simulink model "Isooffboard_SSC"  (R2025b)
settings: Solver=VariableStepAuto  StartTime=0.0  StopTime=0.5  RelTol=1e-3
undefined symbols (not defined in the file): V_ref_isolated
libraries: fl_lib x73, nesl_utility x29, ee_lib x9, simulink x3, eeTransforms x2, batteryecm_lib x1, eeSinusoidalMeasurementV2 x1
(part 2 of 3)

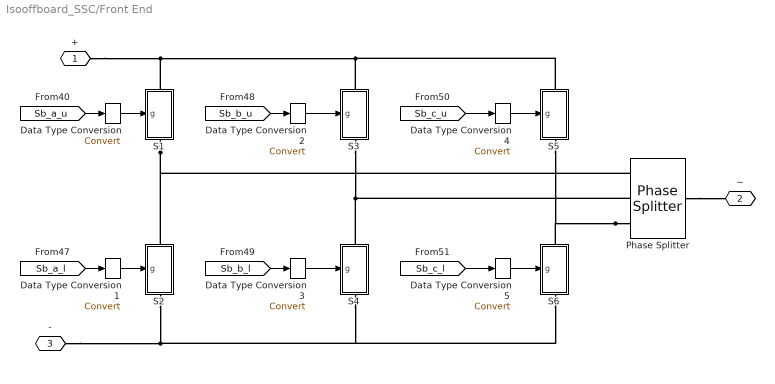
== system Isooffboard_SSC/Front End ==
  Data Type Conversion{,1..5} (6 alike) : DataTypeConversion  SaturateOnIntegerOverflow=off  RndMeth=Floor
  Phase Splitter : ee_lib/Connectors & References/Phase Splitter
  S1 : Subsystem
      settings: PortSchema="{\"entries\":[{\"content\":{\"sides\":[{\"content\":{\"connectorIds\":[\"In1\"]},\"type\":\"ConnectorPlacement.EquallySpacedRectSide\",\"uuid\":\"4868c43b-8f86-4e2f-a4da-367c2e17d6e4\"},{\"content\":{\"side\":\"RIGHT\"},\"type\":\"ConnectorPlacement.EquallySpacedRectSide\",\"uuid\":\"ebe9b5ec-833b-4a08-98e5-ff684cd7afcb\"},{\"content\":{\"connectorIds\":[\"LConn1\"],\"side\":\"TOP\"},\"type\":\"ConnectorPlacement.EquallySpacedRectSide\",\"uuid\":\"c72df866-8baa-41a8-9bb1-42a4a1fdee71\"},{\"content\":{\"connectorIds\":[\"RConn1\"],\"side\":\"BOTTOM\"},\"type\":\"ConnectorPlacement.EquallySpacedRectSide\",\"uuid\":\"3a9867c5-1563-48cb-a4f4-92deec85fd3d\"}]},\"type\":\"ConnectorPlacement.EquallySpacedConnector\",\"uuid\":\"206e0d7b-1d35-45e7-9c4c-8a6f9fe9dc79\"}],\"packageUris\":[\"http://schema.mathworks.com/mf0/Connector/R2020b\"],\"version\":\"1.0\"}"
  S2 : Subsystem
      settings: PortSchema="{\"entries\":[{\"content\":{\"sides\":[{\"content\":{\"connectorIds\":[\"In1\"]},\"type\":\"ConnectorPlacement.EquallySpacedRectSide\",\"uuid\":\"4868c43b-8f86-4e2f-a4da-367c2e17d6e4\"},{\"content\":{\"side\":\"RIGHT\"},\"type\":\"ConnectorPlacement.EquallySpacedRectSide\",\"uuid\":\"ebe9b5ec-833b-4a08-98e5-ff684cd7afcb\"},{\"content\":{\"connectorIds\":[\"LConn1\"],\"side\":\"TOP\"},\"type\":\"ConnectorPlacement.EquallySpacedRectSide\",\"uuid\":\"c72df866-8baa-41a8-9bb1-42a4a1fdee71\"},{\"content\":{\"connectorIds\":[\"RConn1\"],\"side\":\"BOTTOM\"},\"type\":\"ConnectorPlacement.EquallySpacedRectSide\",\"uuid\":\"3a9867c5-1563-48cb-a4f4-92deec85fd3d\"}]},\"type\":\"ConnectorPlacement.EquallySpacedConnector\",\"uuid\":\"206e0d7b-1d35-45e7-9c4c-8a6f9fe9dc79\"}],\"packageUris\":[\"http://schema.mathworks.com/mf0/Connector/R2020b\"],\"version\":\"1.0\"}"
  S3 : Subsystem
      settings: PortSchema="{\"entries\":[{\"content\":{\"sides\":[{\"content\":{\"connectorIds\":[\"In1\"]},\"type\":\"ConnectorPlacement.EquallySpacedRectSide\",\"uuid\":\"4868c43b-8f86-4e2f-a4da-367c2e17d6e4\"},{\"content\":{\"side\":\"RIGHT\"},\"type\":\"ConnectorPlacement.EquallySpacedRectSide\",\"uuid\":\"ebe9b5ec-833b-4a08-98e5-ff684cd7afcb\"},{\"content\":{\"connectorIds\":[\"LConn1\"],\"side\":\"TOP\"},\"type\":\"ConnectorPlacement.EquallySpacedRectSide\",\"uuid\":\"c72df866-8baa-41a8-9bb1-42a4a1fdee71\"},{\"content\":{\"connectorIds\":[\"RConn1\"],\"side\":\"BOTTOM\"},\"type\":\"ConnectorPlacement.EquallySpacedRectSide\",\"uuid\":\"3a9867c5-1563-48cb-a4f4-92deec85fd3d\"}]},\"type\":\"ConnectorPlacement.EquallySpacedConnector\",\"uuid\":\"206e0d7b-1d35-45e7-9c4c-8a6f9fe9dc79\"}],\"packageUris\":[\"http://schema.mathworks.com/mf0/Connector/R2020b\"],\"version\":\"1.0\"}"
  S4 : Subsystem
      settings: PortSchema="{\"entries\":[{\"content\":{\"sides\":[{\"content\":{\"connectorIds\":[\"In1\"]},\"type\":\"ConnectorPlacement.EquallySpacedRectSide\",\"uuid\":\"4868c43b-8f86-4e2f-a4da-367c2e17d6e4\"},{\"content\":{\"side\":\"RIGHT\"},\"type\":\"ConnectorPlacement.EquallySpacedRectSide\",\"uuid\":\"ebe9b5ec-833b-4a08-98e5-ff684cd7afcb\"},{\"content\":{\"connectorIds\":[\"LConn1\"],\"side\":\"TOP\"},\"type\":\"ConnectorPlacement.EquallySpacedRectSide\",\"uuid\":\"c72df866-8baa-41a8-9bb1-42a4a1fdee71\"},{\"content\":{\"connectorIds\":[\"RConn1\"],\"side\":\"BOTTOM\"},\"type\":\"ConnectorPlacement.EquallySpacedRectSide\",\"uuid\":\"3a9867c5-1563-48cb-a4f4-92deec85fd3d\"}]},\"type\":\"ConnectorPlacement.EquallySpacedConnector\",\"uuid\":\"206e0d7b-1d35-45e7-9c4c-8a6f9fe9dc79\"}],\"packageUris\":[\"http://schema.mathworks.com/mf0/Connector/R2020b\"],\"version\":\"1.0\"}"
  S5 : Subsystem
      settings: PortSchema="{\"entries\":[{\"content\":{\"sides\":[{\"content\":{\"connectorIds\":[\"In1\"]},\"type\":\"ConnectorPlacement.EquallySpacedRectSide\",\"uuid\":\"4868c43b-8f86-4e2f-a4da-367c2e17d6e4\"},{\"content\":{\"side\":\"RIGHT\"},\"type\":\"ConnectorPlacement.EquallySpacedRectSide\",\"uuid\":\"ebe9b5ec-833b-4a08-98e5-ff684cd7afcb\"},{\"content\":{\"connectorIds\":[\"LConn1\"],\"side\":\"TOP\"},\"type\":\"ConnectorPlacement.EquallySpacedRectSide\",\"uuid\":\"c72df866-8baa-41a8-9bb1-42a4a1fdee71\"},{\"content\":{\"connectorIds\":[\"RConn1\"],\"side\":\"BOTTOM\"},\"type\":\"ConnectorPlacement.EquallySpacedRectSide\",\"uuid\":\"3a9867c5-1563-48cb-a4f4-92deec85fd3d\"}]},\"type\":\"ConnectorPlacement.EquallySpacedConnector\",\"uuid\":\"206e0d7b-1d35-45e7-9c4c-8a6f9fe9dc79\"}],\"packageUris\":[\"http://schema.mathworks.com/mf0/Connector/R2020b\"],\"version\":\"1.0\"}"
  S6 : Subsystem
      settings: PortSchema="{\"entries\":[{\"content\":{\"sides\":[{\"content\":{\"connectorIds\":[\"In1\"]},\"type\":\"ConnectorPlacement.EquallySpacedRectSide\",\"uuid\":\"4868c43b-8f86-4e2f-a4da-367c2e17d6e4\"},{\"content\":{\"side\":\"RIGHT\"},\"type\":\"ConnectorPlacement.EquallySpacedRectSide\",\"uuid\":\"ebe9b5ec-833b-4a08-98e5-ff684cd7afcb\"},{\"content\":{\"connectorIds\":[\"LConn1\"],\"side\":\"TOP\"},\"type\":\"ConnectorPlacement.EquallySpacedRectSide\",\"uuid\":\"c72df866-8baa-41a8-9bb1-42a4a1fdee71\"},{\"content\":{\"connectorIds\":[\"RConn1\"],\"side\":\"BOTTOM\"},\"type\":\"ConnectorPlacement.EquallySpacedRectSide\",\"uuid\":\"3a9867c5-1563-48cb-a4f4-92deec85fd3d\"}]},\"type\":\"ConnectorPlacement.EquallySpacedConnector\",\"uuid\":\"206e0d7b-1d35-45e7-9c4c-8a6f9fe9dc79\"}],\"packageUris\":[\"http://schema.mathworks.com/mf0/Connector/R2020b\"],\"version\":\"1.0\"}"
  + : PMIOPort  Side=Right
  "~ " : PMIOPort  Port=2  Side=Left
  - : PMIOPort  Port=3  Side=Right
  wires:
  [Sb_c_l] -> Data Type Conversion5/1
  [Sb_b_l] -> Data Type Conversion3/1
  [Sb_a_l] -> Data Type Conversion1/1
  [Sb_a_u] -> Data Type Conversion/1
  [Sb_c_u] -> Data Type Conversion4/1
  [Sb_b_u] -> Data Type Conversion2/1
  Data Type Conversion/1 -> S1/1(g)
  Data Type Conversion1/1 -> S2/1(g)
  Data Type Conversion2/1 -> S3/1(g)
  Data Type Conversion3/1 -> S4/1(g)
  Data Type Conversion4/1 -> S5/1(g)
  Data Type Conversion5/1 -> S6/1(g)
  connections:
  S6/RConn1 -- S4/RConn1 -- S2/RConn1 -- -/RConn1
  S1/LConn1 -- S5/LConn1 -- S3/LConn1 -- +/RConn1
  Phase Splitter/RConn3 -- S6/LConn1 -- S5/RConn1
  Phase Splitter/RConn2 -- S4/LConn1 -- S3/RConn1
  S1/RConn1 -- S2/LConn1 -- Phase Splitter/RConn1
  Phase Splitter/LConn1 -- "~ "/RConn1

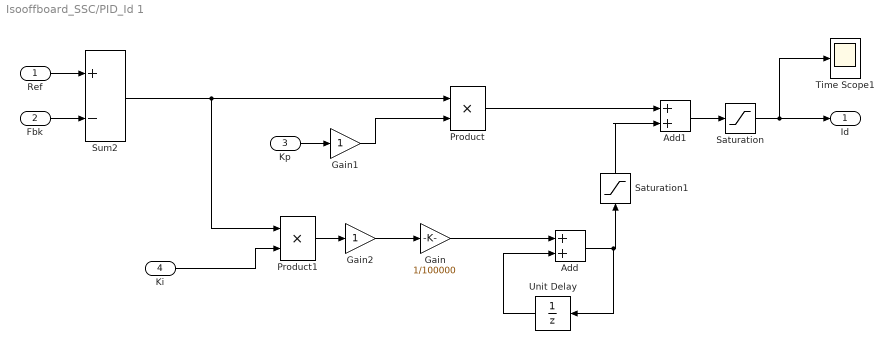
== system Isooffboard_SSC/PID_Id 1 ==
  Ref : Inport
  Fbk : Inport  Port=2
  Kp : Inport  Port=3
  Ki : Inport  Port=4
  Add : Sum
  Add1 : Sum
  Gain : Gain  Gain=1/100000
  Gain1 : Gain
  Gain2 : Gain
  Product : Product  OutDataTypeStr=Inherit: Same as first input
  Product1 : Product  OutDataTypeStr=Inherit: Same as first input
  Saturation : Saturate  UpperLimit=200  LowerLimit=-200  LinearizeAsGain=off  ZeroCross=off
  Saturation1 : Saturate  UpperLimit=200  LowerLimit=-200  LinearizeAsGain=off  ZeroCross=off
  Sum2 : Sum  Inputs=+-
  Time Scope1 : Scope
      settings: TimeUnits=Metric (based on Time Span)  ActiveDisplayYMinimum=-250  ActiveDisplayYMaximum=250  YLabel=Amplitude  DataLoggingVariableName=ScopeData5
  Unit Delay : UnitDelay  SampleTime=-1  HasFrameUpgradeWarning=on
  Id : Outport
  wires:
  Sum2/1 -> Product1/1, Product/1
  Fbk/1 -> Sum2/2
  Ref/1 -> Sum2/1
  Product1/1 -> Gain2/1
  Add/1 -> Unit Delay/1, Saturation1/1
  Product/1 -> Add1/1
  Gain/1 -> Add/1
  Unit Delay/1 -> Add/2
  Kp/1 -> Gain1/1
  Ki/1 -> Product1/2
  Gain1/1 -> Product/2
  Gain2/1 -> Gain/1
  Add1/1 -> Saturation/1
  Saturation/1 -> Time Scope1/1, Id/1
  Saturation1/1 -> Add1/2

== system Isooffboard_SSC/PID_Id 2 ==
  Ref : Inport
  Fbk : Inport  Port=2
  Kp : Inport  Port=3
  Ki : Inport  Port=4
  Add : Sum
  Add1 : Sum
  Gain : Gain  Gain=1/100000
  Product : Product  OutDataTypeStr=Inherit: Same as first input
  Product1 : Product  OutDataTypeStr=Inherit: Same as first input
  Saturation : Saturate  UpperLimit=900  LowerLimit=-900  LinearizeAsGain=off  ZeroCross=off
  Saturation1 : Saturate  UpperLimit=900  LowerLimit=-900  ZeroCross=off
  Sum2 : Sum  Inputs=+-
  Time Scope1 : Scope
      settings: TimeUnits=Metric (based on Time Span)  ActiveDisplayYMinimum=-1125  ActiveDisplayYMaximum=1125  YLabel=Amplitude  DataLoggingVariableName=ScopeData5
  Unit Delay : UnitDelay  SampleTime=-1  HasFrameUpgradeWarning=on
  Ud : Outport
  wires:
  Add1/1 -> Saturation/1
  Sum2/1 -> Product1/1, Product/1
  Fbk/1 -> Sum2/2
  Ref/1 -> Sum2/1
  Kp/1 -> Product/2
  Ki/1 -> Product1/2
  Product1/1 -> Gain/1
  Add/1 -> Unit Delay/1, Saturation1/1
  Product/1 -> Add1/1
  Saturation/1 -> Time Scope1/1, Ud/1
  Gain/1 -> Add/1
  Unit Delay/1 -> Add/2
  Saturation1/1 -> Add1/2

== system Isooffboard_SSC/PID_Iq 3 ==
  Ref : Inport
  Fbk : Inport  Port=2
  Kp : Inport  Port=3
  Ki : Inport  Port=4
  Add : Sum
  Add1 : Sum
  Gain : Gain  Gain=1/100000
  Product : Product  OutDataTypeStr=Inherit: Same as first input
  Product1 : Product  OutDataTypeStr=Inherit: Same as first input
  Saturation : Saturate  UpperLimit=900  LowerLimit=-900  LinearizeAsGain=off  ZeroCross=off
  Saturation1 : Saturate  UpperLimit=900  LowerLimit=-900  LinearizeAsGain=off  ZeroCross=off
  Sum2 : Sum  Inputs=+-
  Time Scope1 : Scope
      settings: TimeUnits=Metric (based on Time Span)  ActiveDisplayYMinimum=-295.24637  ActiveDisplayYMaximum=1032.80515  YLabel=Amplitude  DataLoggingVariableName=ScopeData6
  Unit Delay : UnitDelay  SampleTime=-1  HasFrameUpgradeWarning=on
  Uq : Outport
  wires:
  Add1/1 -> Saturation/1
  Sum2/1 -> Product1/1, Product/1
  Fbk/1 -> Sum2/2
  Ref/1 -> Sum2/1
  Kp/1 -> Product/2
  Ki/1 -> Product1/2
  Product1/1 -> Gain/1
  Add/1 -> Unit Delay/1, Saturation1/1
  Product/1 -> Add1/1
  Gain/1 -> Add/1
  Unit Delay/1 -> Add/2
  Saturation/1 -> Time Scope1/1, Uq/1
  Saturation1/1 -> Add1/2

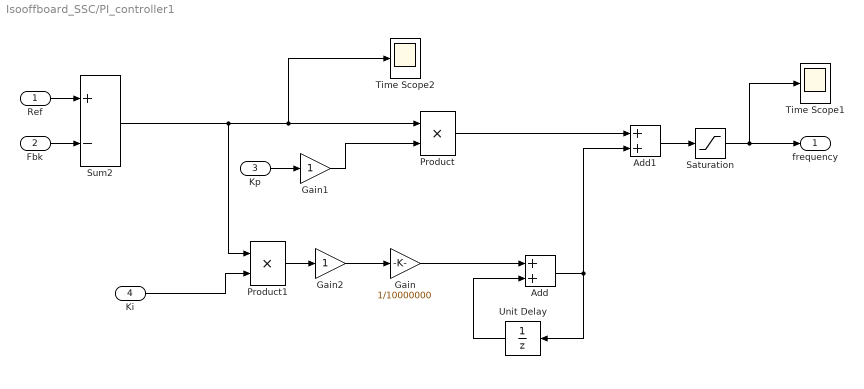
== system Isooffboard_SSC/PI_controller1 ==
  Ref : Inport
  Fbk : Inport  Port=2
  Kp : Inport  Port=3
  Ki : Inport  Port=4
  Add : Sum
  Add1 : Sum
  Gain : Gain  Gain=1/10000000
  Gain1 : Gain
  Gain2 : Gain
  Product : Product  OutDataTypeStr=Inherit: Same as first input
  Product1 : Product  OutDataTypeStr=Inherit: Same as first input
  Saturation : Saturate  UpperLimit=1  LowerLimit=0.5  LinearizeAsGain=off  ZeroCross=off
  Sum2 : Sum  Inputs=+-
  Time Scope1 : Scope
      settings: TimeUnits=Metric (based on Time Span)  ActiveDisplayYMinimum=0.4375  ActiveDisplayYMaximum=1.0625  YLabel=Amplitude  DataLoggingVariableName=ScopeData5
  Time Scope2 : Scope
      settings: TimeUnits=Metric (based on Time Span)  ActiveDisplayYMinimum=-48.22028  ActiveDisplayYMaximum=227.58003  YLabel=Amplitude  DataLoggingVariableName=ScopeData6
  Unit Delay : UnitDelay  InitialCondition=0.9  SampleTime=-1  HasFrameUpgradeWarning=on
  frequency : Outport
  wires:
  Fbk/1 -> Sum2/2
  Ref/1 -> Sum2/1
  Product1/1 -> Gain2/1
  Add/1 -> Unit Delay/1, Add1/2
  Product/1 -> Add1/1
  Gain/1 -> Add/1
  Unit Delay/1 -> Add/2
  Ki/1 -> Product1/2
  Gain2/1 -> Gain/1
  Add1/1 -> Saturation/1
  Saturation/1 -> Time Scope1/1, frequency/1
  Kp/1 -> Gain1/1
  Gain1/1 -> Product/2
  Sum2/1 -> Product1/1, Time Scope2/1, Product/1

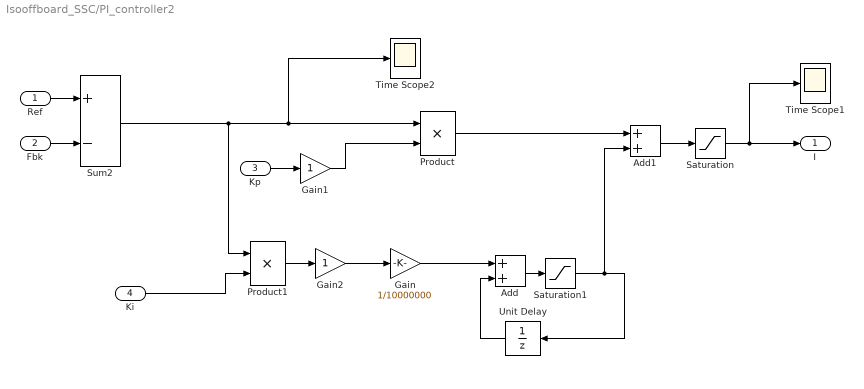
== system Isooffboard_SSC/PI_controller2 ==
  Ref : Inport
  Fbk : Inport  Port=2
  Kp : Inport  Port=3
  Ki : Inport  Port=4
  Add : Sum
  Add1 : Sum
  Gain : Gain  Gain=1/10000000
  Gain1 : Gain
  Gain2 : Gain
  Product : Product  OutDataTypeStr=Inherit: Same as first input
  Product1 : Product  OutDataTypeStr=Inherit: Same as first input
  Saturation : Saturate  UpperLimit=50  LowerLimit=-50  LinearizeAsGain=off  ZeroCross=off
  Saturation1 : Saturate  UpperLimit=50  LowerLimit=-50  LinearizeAsGain=off  ZeroCross=off
  Sum2 : Sum  Inputs=+-
  Time Scope1 : Scope
      settings: TimeUnits=Metric (based on Time Span)  ActiveDisplayYMinimum=-55.24132  ActiveDisplayYMaximum=61.69348  YLabel=Amplitude  DataLoggingVariableName=ScopeData5
  Time Scope2 : Scope
      settings: TimeUnits=Metric (based on Time Span)  ActiveDisplayYMinimum=-48.22028  ActiveDisplayYMaximum=227.58003  YLabel=Amplitude  DataLoggingVariableName=ScopeData6
  Unit Delay : UnitDelay  InitialCondition=0.9  SampleTime=-1  HasFrameUpgradeWarning=on
  I : Outport
  wires:
  Fbk/1 -> Sum2/2
  Ref/1 -> Sum2/1
  Product1/1 -> Gain2/1
  Product/1 -> Add1/1
  Gain/1 -> Add/1
  Unit Delay/1 -> Add/2
  Ki/1 -> Product1/2
  Gain2/1 -> Gain/1
  Add1/1 -> Saturation/1
  Saturation/1 -> Time Scope1/1, I/1
  Kp/1 -> Gain1/1
  Gain1/1 -> Product/2
  Sum2/1 -> Product1/1, Time Scope2/1, Product/1
  Add/1 -> Saturation1/1
  Saturation1/1 -> Add1/2, Unit Delay/1

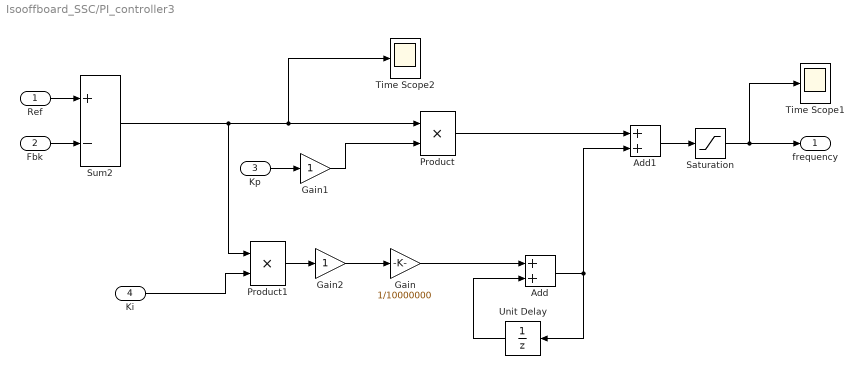
== system Isooffboard_SSC/PI_controller3 ==
  Ref : Inport
  Fbk : Inport  Port=2
  Kp : Inport  Port=3
  Ki : Inport  Port=4
  Add : Sum
  Add1 : Sum
  Gain : Gain  Gain=1/10000000
  Gain1 : Gain
  Gain2 : Gain
  Product : Product  OutDataTypeStr=Inherit: Same as first input
  Product1 : Product  OutDataTypeStr=Inherit: Same as first input
  Saturation : Saturate  UpperLimit=1  LowerLimit=0.5  LinearizeAsGain=off  ZeroCross=off
  Sum2 : Sum  Inputs=+-
  Time Scope1 : Scope
      settings: TimeUnits=Metric (based on Time Span)  ActiveDisplayYMinimum=0.4375  ActiveDisplayYMaximum=1.0625  YLabel=Amplitude  DataLoggingVariableName=ScopeData5
  Time Scope2 : Scope
      settings: TimeUnits=Metric (based on Time Span)  ActiveDisplayYMinimum=-48.22028  ActiveDisplayYMaximum=227.58003  YLabel=Amplitude  DataLoggingVariableName=ScopeData6
  Unit Delay : UnitDelay  InitialCondition=0.9  SampleTime=-1  HasFrameUpgradeWarning=on
  frequency : Outport
  wires:
  Fbk/1 -> Sum2/2
  Ref/1 -> Sum2/1
  Product1/1 -> Gain2/1
  Add/1 -> Unit Delay/1, Add1/2
  Product/1 -> Add1/1
  Gain/1 -> Add/1
  Unit Delay/1 -> Add/2
  Ki/1 -> Product1/2
  Gain2/1 -> Gain/1
  Add1/1 -> Saturation/1
  Saturation/1 -> Time Scope1/1, frequency/1
  Kp/1 -> Gain1/1
  Gain1/1 -> Product/2
  Sum2/1 -> Product1/1, Time Scope2/1, Product/1

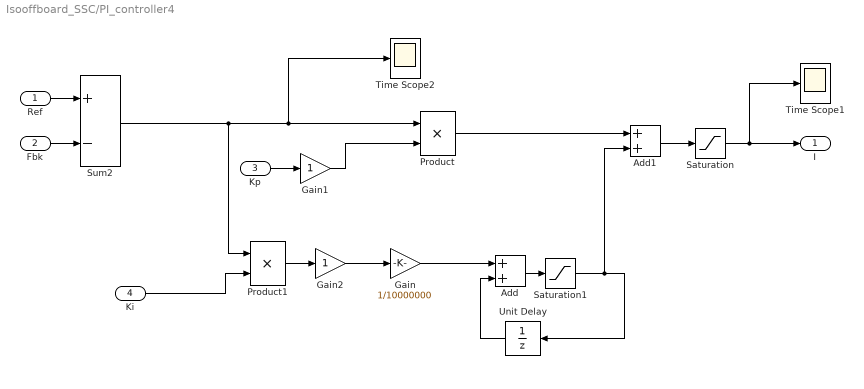
== system Isooffboard_SSC/PI_controller4 ==
  Ref : Inport
  Fbk : Inport  Port=2
  Kp : Inport  Port=3
  Ki : Inport  Port=4
  Add : Sum
  Add1 : Sum
  Gain : Gain  Gain=1/10000000
  Gain1 : Gain
  Gain2 : Gain
  Product : Product  OutDataTypeStr=Inherit: Same as first input
  Product1 : Product  OutDataTypeStr=Inherit: Same as first input
  Saturation : Saturate  UpperLimit=50  LowerLimit=-50  LinearizeAsGain=off  ZeroCross=off
  Saturation1 : Saturate  UpperLimit=50  LowerLimit=-50  LinearizeAsGain=off  ZeroCross=off
  Sum2 : Sum  Inputs=+-
  Time Scope1 : Scope
      settings: TimeUnits=Metric (based on Time Span)  ActiveDisplayYMinimum=-55.24132  ActiveDisplayYMaximum=61.69348  YLabel=Amplitude  DataLoggingVariableName=ScopeData5
  Time Scope2 : Scope
      settings: TimeUnits=Metric (based on Time Span)  ActiveDisplayYMinimum=-48.22028  ActiveDisplayYMaximum=227.58003  YLabel=Amplitude  DataLoggingVariableName=ScopeData6
  Unit Delay : UnitDelay  InitialCondition=0.9  SampleTime=-1  HasFrameUpgradeWarning=on
  I : Outport
  wires:
  Fbk/1 -> Sum2/2
  Ref/1 -> Sum2/1
  Product1/1 -> Gain2/1
  Product/1 -> Add1/1
  Gain/1 -> Add/1
  Unit Delay/1 -> Add/2
  Ki/1 -> Product1/2
  Gain2/1 -> Gain/1
  Add1/1 -> Saturation/1
  Saturation/1 -> Time Scope1/1, I/1
  Kp/1 -> Gain1/1
  Gain1/1 -> Product/2
  Sum2/1 -> Product1/1, Time Scope2/1, Product/1
  Add/1 -> Saturation1/1
  Saturation1/1 -> Add1/2, Unit Delay/1

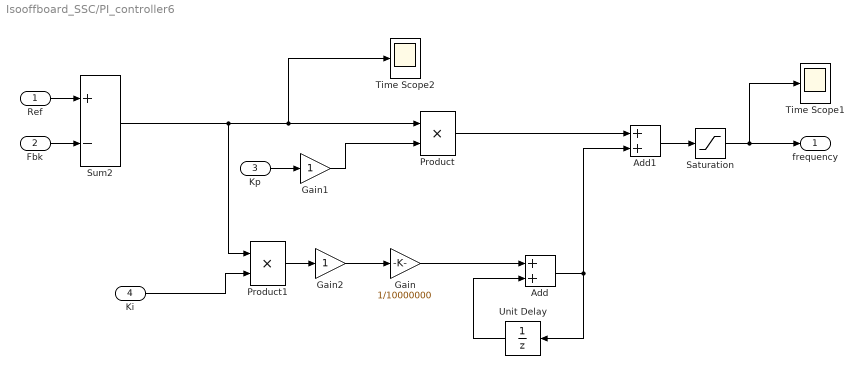
== system Isooffboard_SSC/PI_controller6 ==
  Ref : Inport
  Fbk : Inport  Port=2
  Kp : Inport  Port=3
  Ki : Inport  Port=4
  Add : Sum
  Add1 : Sum
  Gain : Gain  Gain=1/10000000
  Gain1 : Gain
  Gain2 : Gain
  Product : Product  OutDataTypeStr=Inherit: Same as first input
  Product1 : Product  OutDataTypeStr=Inherit: Same as first input
  Saturation : Saturate  UpperLimit=1  LowerLimit=0.5  LinearizeAsGain=off  ZeroCross=off
  Sum2 : Sum  Inputs=+-
  Time Scope1 : Scope
      settings: TimeUnits=Metric (based on Time Span)  ActiveDisplayYMinimum=0.4375  ActiveDisplayYMaximum=1.0625  YLabel=Amplitude  DataLoggingVariableName=ScopeData5
  Time Scope2 : Scope
      settings: TimeUnits=Metric (based on Time Span)  ActiveDisplayYMinimum=-48.22028  ActiveDisplayYMaximum=227.58003  YLabel=Amplitude  DataLoggingVariableName=ScopeData6
  Unit Delay : UnitDelay  InitialCondition=0.9  SampleTime=-1  HasFrameUpgradeWarning=on
  frequency : Outport
  wires:
  Fbk/1 -> Sum2/2
  Ref/1 -> Sum2/1
  Product1/1 -> Gain2/1
  Add/1 -> Unit Delay/1, Add1/2
  Product/1 -> Add1/1
  Gain/1 -> Add/1
  Unit Delay/1 -> Add/2
  Ki/1 -> Product1/2
  Gain2/1 -> Gain/1
  Add1/1 -> Saturation/1
  Saturation/1 -> Time Scope1/1, frequency/1
  Kp/1 -> Gain1/1
  Gain1/1 -> Product/2
  Sum2/1 -> Product1/1, Time Scope2/1, Product/1

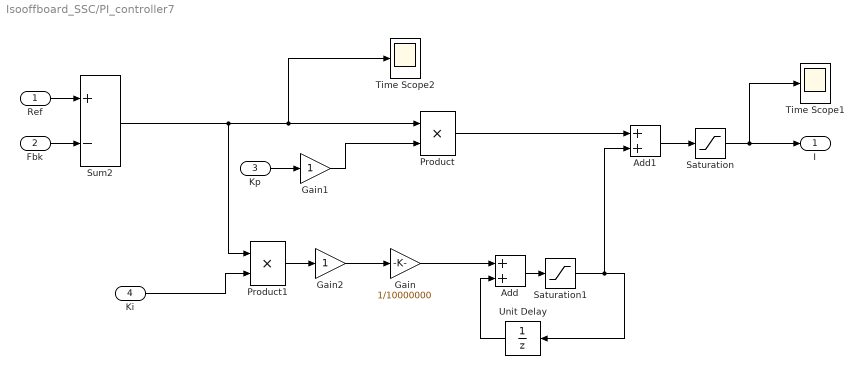
== system Isooffboard_SSC/PI_controller7 ==
  Ref : Inport
  Fbk : Inport  Port=2
  Kp : Inport  Port=3
  Ki : Inport  Port=4
  Add : Sum
  Add1 : Sum
  Gain : Gain  Gain=1/10000000
  Gain1 : Gain
  Gain2 : Gain
  Product : Product  OutDataTypeStr=Inherit: Same as first input
  Product1 : Product  OutDataTypeStr=Inherit: Same as first input
  Saturation : Saturate  UpperLimit=50  LowerLimit=-50  LinearizeAsGain=off  ZeroCross=off
  Saturation1 : Saturate  UpperLimit=50  LowerLimit=-50  LinearizeAsGain=off  ZeroCross=off
  Sum2 : Sum  Inputs=+-
  Time Scope1 : Scope
      settings: TimeUnits=Metric (based on Time Span)  ActiveDisplayYMinimum=-55.24132  ActiveDisplayYMaximum=61.69348  YLabel=Amplitude  DataLoggingVariableName=ScopeData5
  Time Scope2 : Scope
      settings: TimeUnits=Metric (based on Time Span)  ActiveDisplayYMinimum=-48.22028  ActiveDisplayYMaximum=227.58003  YLabel=Amplitude  DataLoggingVariableName=ScopeData6
  Unit Delay : UnitDelay  InitialCondition=0.9  SampleTime=-1  HasFrameUpgradeWarning=on
  I : Outport
  wires:
  Fbk/1 -> Sum2/2
  Ref/1 -> Sum2/1
  Product1/1 -> Gain2/1
  Product/1 -> Add1/1
  Gain/1 -> Add/1
  Unit Delay/1 -> Add/2
  Ki/1 -> Product1/2
  Gain2/1 -> Gain/1
  Add1/1 -> Saturation/1
  Saturation/1 -> Time Scope1/1, I/1
  Kp/1 -> Gain1/1
  Gain1/1 -> Product/2
  Sum2/1 -> Product1/1, Time Scope2/1, Product/1
  Add/1 -> Saturation1/1
  Saturation1/1 -> Add1/2, Unit Delay/1

== system Isooffboard_SSC/Subsystem ==
  PS-Simulink Converter2 : nesl_utility/PS-Simulink Converter  PhysicalDomain=network_engine_domain  SubClassName=ps_output  LeftPortType=input  RightPortType=output  PseudoPeriodic=off  Frequencies=[]  VectorFormat=inherit  Unit=inherit  AffineConversion=off
  Unit Delay1 : UnitDelay  SampleTime=-1  HasFrameUpgradeWarning=on
  Voltage Sensor : fl_lib/Electrical/Electrical Sensors/Voltage Sensor
  + : PMIOPort  Side=Left
  - : PMIOPort  Port=2  Side=Right
  V : Outport
  wires:
  PS-Simulink Converter2/1 -> Unit Delay1/1
  Unit Delay1/1 -> V/1
  connections:
  Voltage Sensor/LConn1 -- +/RConn1
  PS-Simulink Converter2/LConn1 -- Voltage Sensor/RConn1
  Voltage Sensor/RConn2 -- -/RConn1

== system Isooffboard_SSC/Subsystem1 ==
  Va : Inport
  Va1 : Inport  Port=2
  Add1 : Sum
  Constant8 : Constant  Value=0.5
  Divide : Product  Inputs=*/
  Logical Operator1 : Logic  Operator=NOT  AllPortsSameDT=off  OutDataTypeStr=boolean
  Relational Operator : RelationalOperator  OutDataTypeStr=boolean  ZeroCross=off  InputSameDT=off
  Repeating Sequence : simulink/Sources/Repeating Sequence  rep_seq_t=[0 1/30000/2 1/30000]  rep_seq_y=[0 1 0]
  Scope1 : Scope  NumInputPorts=2
      settings: ActiveDisplayYMinimum=-0.12496  ActiveDisplayYMaximum=1.12466  DataLoggingVariableName=ScopeData3
  Scope2 : Scope  NumInputPorts=2
      settings: ActiveDisplayYMinimum=-0.59999  ActiveDisplayYMaximum=3.15933
  Scope3 : Scope  NumInputPorts=2
      settings: ActiveDisplayYMinimum=-0.125  ActiveDisplayYMaximum=1.125  DataLoggingVariableName=ScopeData2
  Vcomp*2 : Constant  Value=1200
  A : Outport
  A' : Outport  Port=2
  wires:
  Va/1 -> Divide/1
  Divide/1 -> Add1/1
  Add1/1 -> Scope2/1, Relational Operator/2
  Constant8/1 -> Add1/2
  Repeating Sequence/1 -> Scope1/1, Relational Operator/1
  Logical Operator1/1 -> Scope3/1, A/1
  Relational Operator/1 -> Scope3/2, A'/1, Logical Operator1/1
  Va1/1 -> Divide/2

== system Isooffboard_SSC/Subsystem2 ==
  Vb : Inport
  Va : Inport  Port=2
  Add1 : Sum
  Constant8 : Constant  Value=0.5
  Divide : Product  Inputs=*/
  Logical Operator1 : Logic  Operator=NOT  AllPortsSameDT=off  OutDataTypeStr=boolean
  Relational Operator : RelationalOperator  OutDataTypeStr=boolean  ZeroCross=off  InputSameDT=off
  Repeating Sequence : simulink/Sources/Repeating Sequence  rep_seq_t=[0 1/30000/2 1/30000]  rep_seq_y=[0 1 0]
  Scope1 : Scope  NumInputPorts=2
      settings: ActiveDisplayYMinimum=-0.125  ActiveDisplayYMaximum=1.125  DataLoggingVariableName=ScopeData3
  Scope4 : Scope  NumInputPorts=2
      settings: ActiveDisplayYMinimum=-500  ActiveDisplayYMaximum=500  DataLoggingVariableName=ScopeData3
  Vcomp*2 : Constant  Value=1200
  B : Outport
  B' : Outport  Port=2
  wires:
  Vb/1 -> Divide/1
  Divide/1 -> Add1/1
  Add1/1 -> Relational Operator/2, Scope4/2
  Constant8/1 -> Add1/2
  Repeating Sequence/1 -> Scope1/1, Relational Operator/1
  Logical Operator1/1 -> B/1
  Relational Operator/1 -> B'/1, Logical Operator1/1
  Va/1 -> Divide/2

== system Isooffboard_SSC/Subsystem3 ==
  fre : Inport
  Constant8 : Constant  Value=0.5
  Logical Operator1 : Logic  Operator=NOT  AllPortsSameDT=off  OutDataTypeStr=boolean
  MATLAB Function : MATLAB Function  TreatAsAtomicUnit=on
  Relational Operator : RelationalOperator  OutDataTypeStr=boolean  ZeroCross=off  InputSameDT=off
  Scope1 : Scope  NumInputPorts=2
      settings: ActiveDisplayYMinimum=-0.125  ActiveDisplayYMaximum=1.125  DataLoggingVariableName=ScopeData3
  Scope2 : Scope  NumInputPorts=2
      settings: ActiveDisplayYMinimum=0.9  ActiveDisplayYMaximum=1.1
  Scope3 : Scope  NumInputPorts=2
      settings: ActiveDisplayYMinimum=0.40709  ActiveDisplayYMaximum=0.54786  DataLoggingVariableName=ScopeData2
  A : Outport
  A' : Outport  Port=2
  wires:
  Constant8/1 -> Scope2/1, Relational Operator/2
  MATLAB Function/1(y) -> Scope1/1, Relational Operator/1
  Logical Operator1/1 -> Scope3/1, A/1
  Relational Operator/1 -> Scope3/2, A'/1, Logical Operator1/1
  fre/1 -> MATLAB Function/1(u)

== system Isooffboard_SSC/Subsystem4 ==
  Vc : Inport
  Va : Inport  Port=2
  Add1 : Sum
  Constant8 : Constant  Value=0.5
  Divide : Product  Inputs=*/
  Logical Operator1 : Logic  Operator=NOT  AllPortsSameDT=off  OutDataTypeStr=boolean
  Relational Operator : RelationalOperator  OutDataTypeStr=boolean  ZeroCross=off  InputSameDT=off
  Repeating Sequence : simulink/Sources/Repeating Sequence  rep_seq_t=[0 1/30000/2 1/30000]  rep_seq_y=[0 1 0]
  Scope1 : Scope  NumInputPorts=2
      settings: ActiveDisplayYMinimum=-0.125  ActiveDisplayYMaximum=1.125  DataLoggingVariableName=ScopeData3
  Scope4 : Scope  NumInputPorts=2
      settings: ActiveDisplayYMinimum=-500  ActiveDisplayYMaximum=500  DataLoggingVariableName=ScopeData3
  Vcomp*2 : Constant  Value=1200
  C : Outport
  C' : Outport  Port=2
  wires:
  Vc/1 -> Divide/1
  Divide/1 -> Add1/1
  Add1/1 -> Relational Operator/2, Scope4/2
  Constant8/1 -> Add1/2
  Repeating Sequence/1 -> Scope1/1, Relational Operator/1
  Logical Operator1/1 -> C/1
  Relational Operator/1 -> C'/1, Logical Operator1/1
  Va/1 -> Divide/2

== system Isooffboard_SSC/Subsystem5 ==
  fre : Inport
  Constant8 : Constant  Value=0.5
  Logical Operator1 : Logic  Operator=NOT  AllPortsSameDT=off  OutDataTypeStr=boolean
  MATLAB Function : MATLAB Function  TreatAsAtomicUnit=on
  Relational Operator : RelationalOperator  OutDataTypeStr=boolean  ZeroCross=off  InputSameDT=off
  Scope1 : Scope  NumInputPorts=2
      settings: ActiveDisplayYMinimum=-0.125  ActiveDisplayYMaximum=1.125  DataLoggingVariableName=ScopeData3
  Scope2 : Scope  NumInputPorts=2
      settings: ActiveDisplayYMinimum=0.9  ActiveDisplayYMaximum=1.1
  Scope3 : Scope  NumInputPorts=2
      settings: ActiveDisplayYMinimum=0.40709  ActiveDisplayYMaximum=0.54786  DataLoggingVariableName=ScopeData2
  A : Outport
  A' : Outport  Port=2
  wires:
  Constant8/1 -> Scope2/1, Relational Operator/2
  MATLAB Function/1(y) -> Scope1/1, Relational Operator/1
  Logical Operator1/1 -> Scope3/1, A/1
  Relational Operator/1 -> Scope3/2, A'/1, Logical Operator1/1
  fre/1 -> MATLAB Function/1(u)

== system Isooffboard_SSC/Subsystem6 ==
  PS-Simulink Converter2 : nesl_utility/PS-Simulink Converter  PhysicalDomain=network_engine_domain  SubClassName=ps_output  LeftPortType=input  RightPortType=output  PseudoPeriodic=off  Frequencies=[]  VectorFormat=inherit  Unit=inherit  AffineConversion=off
  Unit Delay1 : UnitDelay  SampleTime=-1  HasFrameUpgradeWarning=on
  Voltage Sensor : fl_lib/Electrical/Electrical Sensors/Voltage Sensor
  + : PMIOPort  Side=Left
  - : PMIOPort  Port=2  Side=Right
  V : Outport
  wires:
  Unit Delay1/1 -> V/1
  PS-Simulink Converter2/1 -> Unit Delay1/1
  connections:
  Voltage Sensor/RConn2 -- -/RConn1
  PS-Simulink Converter2/LConn1 -- Voltage Sensor/RConn1
  Voltage Sensor/LConn1 -- +/RConn1

== system Isooffboard_SSC/Subsystem7 ==
  fre : Inport
  Constant8 : Constant  Value=0.5
  Logical Operator1 : Logic  Operator=NOT  AllPortsSameDT=off  OutDataTypeStr=boolean
  MATLAB Function : MATLAB Function  TreatAsAtomicUnit=on
  Relational Operator : RelationalOperator  OutDataTypeStr=boolean  ZeroCross=off  InputSameDT=off
  Scope1 : Scope  NumInputPorts=2
      settings: ActiveDisplayYMinimum=-0.125  ActiveDisplayYMaximum=1.125  DataLoggingVariableName=ScopeData3
  Scope2 : Scope  NumInputPorts=2
      settings: ActiveDisplayYMinimum=0.9  ActiveDisplayYMaximum=1.1
  Scope3 : Scope  NumInputPorts=2
      settings: ActiveDisplayYMinimum=0.40709  ActiveDisplayYMaximum=0.54786  DataLoggingVariableName=ScopeData2
  A : Outport
  A' : Outport  Port=2
  wires:
  Constant8/1 -> Scope2/1, Relational Operator/2
  MATLAB Function/1(y) -> Scope1/1, Relational Operator/1
  Logical Operator1/1 -> Scope3/1, A/1
  Relational Operator/1 -> Scope3/2, A'/1, Logical Operator1/1
  fre/1 -> MATLAB Function/1(u)

== system Isooffboard_SSC/DAB1/S1 ==
  g : Inport
  Diode : fl_lib/Electrical/Electrical Elements/Diode  Vf=1e-3 V  Ron=1e-2 Ohm  Goff=1e-5 1/Ohm  i_specify=off  i_priority=None  i=0 A  i_nominal_specify=off  i_nominal_value=1  i_nominal_unit=A  v_specify=off  v_priority=None  v=0 V  v_nominal_specify=off  v_nominal_value=1  v_nominal_unit=V
  S1 : fl_lib/Electrical/Electrical Elements/Switch  R_closed=0.1 Ohm  G_open=1e-5 1/Ohm  Threshold=0.5  i_specify=off  i_priority=None  i=0 A  i_nominal_specify=off  i_nominal_value=1  i_nominal_unit=A  v_specify=off  v_priority=None  v=0 V  v_nominal_specify=off  v_nominal_value=1  v_nominal_unit=V
  Simulink-PS Converter : nesl_utility/Simulink-PS Converter  PhysicalDomain=network_engine_domain  SubClassName=ps_input  LeftPortType=input  RightPortType=output  PseudoPeriodic=off  Frequencies=[]  NoiseDistribution=none  NoiseParameters=[]  Unit=1  AffineConversion=off  FilteringAndDerivatives=zero  SimscapeFilterOrder=1  InputFilterTimeConstant=0.001  UdotUserProvided=0
  + : PMIOPort  Side=Left
  - : PMIOPort  Port=2  Side=Right
  wires:
  g/1 -> Simulink-PS Converter/1
  connections:
  S1/RConn2 -- -/RConn1 -- Diode/LConn1
  Diode/RConn1 -- +/RConn1 -- S1/LConn1
  Simulink-PS Converter/RConn1 -- S1/RConn1

== system Isooffboard_SSC/DAB1/S2 ==
  g : Inport
  Diode : fl_lib/Electrical/Electrical Elements/Diode  Vf=1e-3 V  Ron=1e-2 Ohm  Goff=1e-5 1/Ohm  i_specify=off  i_priority=None  i=0 A  i_nominal_specify=off  i_nominal_value=1  i_nominal_unit=A  v_specify=off  v_priority=None  v=0 V  v_nominal_specify=off  v_nominal_value=1  v_nominal_unit=V
  S1 : fl_lib/Electrical/Electrical Elements/Switch  R_closed=0.1 Ohm  G_open=1e-5 1/Ohm  Threshold=0.5  i_specify=off  i_priority=None  i=0 A  i_nominal_specify=off  i_nominal_value=1  i_nominal_unit=A  v_specify=off  v_priority=None  v=0 V  v_nominal_specify=off  v_nominal_value=1  v_nominal_unit=V
  Simulink-PS Converter : nesl_utility/Simulink-PS Converter  PhysicalDomain=network_engine_domain  SubClassName=ps_input  LeftPortType=input  RightPortType=output  PseudoPeriodic=off  Frequencies=[]  NoiseDistribution=none  NoiseParameters=[]  Unit=1  AffineConversion=off  FilteringAndDerivatives=zero  SimscapeFilterOrder=1  InputFilterTimeConstant=0.001  UdotUserProvided=0
  + : PMIOPort  Side=Left
  - : PMIOPort  Port=2  Side=Right
  wires:
  g/1 -> Simulink-PS Converter/1
  connections:
  Simulink-PS Converter/RConn1 -- S1/RConn1
  S1/LConn1 -- +/RConn1 -- Diode/RConn1
  Diode/LConn1 -- -/RConn1 -- S1/RConn2

== system Isooffboard_SSC/DAB1/S3 ==
  g : Inport
  Diode : fl_lib/Electrical/Electrical Elements/Diode  Vf=1e-3 V  Ron=1e-2 Ohm  Goff=1e-5 1/Ohm  i_specify=off  i_priority=None  i=0 A  i_nominal_specify=off  i_nominal_value=1  i_nominal_unit=A  v_specify=off  v_priority=None  v=0 V  v_nominal_specify=off  v_nominal_value=1  v_nominal_unit=V
  S1 : fl_lib/Electrical/Electrical Elements/Switch  R_closed=0.1 Ohm  G_open=1e-5 1/Ohm  Threshold=0.5  i_specify=off  i_priority=None  i=0 A  i_nominal_specify=off  i_nominal_value=1  i_nominal_unit=A  v_specify=off  v_priority=None  v=0 V  v_nominal_specify=off  v_nominal_value=1  v_nominal_unit=V
  Simulink-PS Converter : nesl_utility/Simulink-PS Converter  PhysicalDomain=network_engine_domain  SubClassName=ps_input  LeftPortType=input  RightPortType=output  PseudoPeriodic=off  Frequencies=[]  NoiseDistribution=none  NoiseParameters=[]  Unit=1  AffineConversion=off  FilteringAndDerivatives=zero  SimscapeFilterOrder=1  InputFilterTimeConstant=0.001  UdotUserProvided=0
  + : PMIOPort  Side=Left
  - : PMIOPort  Port=2  Side=Right
  wires:
  g/1 -> Simulink-PS Converter/1
  connections:
  S1/RConn2 -- -/RConn1 -- Diode/LConn1
  Diode/RConn1 -- +/RConn1 -- S1/LConn1
  Simulink-PS Converter/RConn1 -- S1/RConn1

== system Isooffboard_SSC/DAB1/S4 ==
  g : Inport
  Diode : fl_lib/Electrical/Electrical Elements/Diode  Vf=1e-3 V  Ron=1e-2 Ohm  Goff=1e-5 1/Ohm  i_specify=off  i_priority=None  i=0 A  i_nominal_specify=off  i_nominal_value=1  i_nominal_unit=A  v_specify=off  v_priority=None  v=0 V  v_nominal_specify=off  v_nominal_value=1  v_nominal_unit=V
  S1 : fl_lib/Electrical/Electrical Elements/Switch  R_closed=0.1 Ohm  G_open=1e-5 1/Ohm  Threshold=0.5  i_specify=off  i_priority=None  i=0 A  i_nominal_specify=off  i_nominal_value=1  i_nominal_unit=A  v_specify=off  v_priority=None  v=0 V  v_nominal_specify=off  v_nominal_value=1  v_nominal_unit=V
  Simulink-PS Converter : nesl_utility/Simulink-PS Converter  PhysicalDomain=network_engine_domain  SubClassName=ps_input  LeftPortType=input  RightPortType=output  PseudoPeriodic=off  Frequencies=[]  NoiseDistribution=none  NoiseParameters=[]  Unit=1  AffineConversion=off  FilteringAndDerivatives=zero  SimscapeFilterOrder=1  InputFilterTimeConstant=0.001  UdotUserProvided=0
  + : PMIOPort  Side=Left
  - : PMIOPort  Port=2  Side=Right
  wires:
  g/1 -> Simulink-PS Converter/1
  connections:
  Simulink-PS Converter/RConn1 -- S1/RConn1
  S1/LConn1 -- +/RConn1 -- Diode/RConn1
  Diode/LConn1 -- -/RConn1 -- S1/RConn2

== system Isooffboard_SSC/DAB2/S1 ==
  g : Inport
  Diode : fl_lib/Electrical/Electrical Elements/Diode  Vf=1e-3 V  Ron=1e-2 Ohm  Goff=1e-5 1/Ohm  i_specify=off  i_priority=None  i=0 A  i_nominal_specify=off  i_nominal_value=1  i_nominal_unit=A  v_specify=off  v_priority=None  v=0 V  v_nominal_specify=off  v_nominal_value=1  v_nominal_unit=V
  S1 : fl_lib/Electrical/Electrical Elements/Switch  R_closed=0.1 Ohm  G_open=1e-5 1/Ohm  Threshold=0.5  i_specify=off  i_priority=None  i=0 A  i_nominal_specify=off  i_nominal_value=1  i_nominal_unit=A  v_specify=off  v_priority=None  v=0 V  v_nominal_specify=off  v_nominal_value=1  v_nominal_unit=V
  Simulink-PS Converter : nesl_utility/Simulink-PS Converter  PhysicalDomain=network_engine_domain  SubClassName=ps_input  LeftPortType=input  RightPortType=output  PseudoPeriodic=off  Frequencies=[]  NoiseDistribution=none  NoiseParameters=[]  Unit=1  AffineConversion=off  FilteringAndDerivatives=zero  SimscapeFilterOrder=1  InputFilterTimeConstant=0.001  UdotUserProvided=0
  + : PMIOPort  Side=Left
  - : PMIOPort  Port=2  Side=Right
  wires:
  g/1 -> Simulink-PS Converter/1
  connections:
  Simulink-PS Converter/RConn1 -- S1/RConn1
  S1/LConn1 -- +/RConn1 -- Diode/RConn1
  Diode/LConn1 -- -/RConn1 -- S1/RConn2

== system Isooffboard_SSC/DAB2/S2 ==
  g : Inport
  Diode : fl_lib/Electrical/Electrical Elements/Diode  Vf=1e-3 V  Ron=1e-2 Ohm  Goff=1e-5 1/Ohm  i_specify=off  i_priority=None  i=0 A  i_nominal_specify=off  i_nominal_value=1  i_nominal_unit=A  v_specify=off  v_priority=None  v=0 V  v_nominal_specify=off  v_nominal_value=1  v_nominal_unit=V
  S1 : fl_lib/Electrical/Electrical Elements/Switch  R_closed=0.1 Ohm  G_open=1e-5 1/Ohm  Threshold=0.5  i_specify=off  i_priority=None  i=0 A  i_nominal_specify=off  i_nominal_value=1  i_nominal_unit=A  v_specify=off  v_priority=None  v=0 V  v_nominal_specify=off  v_nominal_value=1  v_nominal_unit=V
  Simulink-PS Converter : nesl_utility/Simulink-PS Converter  PhysicalDomain=network_engine_domain  SubClassName=ps_input  LeftPortType=input  RightPortType=output  PseudoPeriodic=off  Frequencies=[]  NoiseDistribution=none  NoiseParameters=[]  Unit=1  AffineConversion=off  FilteringAndDerivatives=zero  SimscapeFilterOrder=1  InputFilterTimeConstant=0.001  UdotUserProvided=0
  + : PMIOPort  Side=Left
  - : PMIOPort  Port=2  Side=Right
  wires:
  g/1 -> Simulink-PS Converter/1
  connections:
  S1/RConn2 -- -/RConn1 -- Diode/LConn1
  Diode/RConn1 -- +/RConn1 -- S1/LConn1
  Simulink-PS Converter/RConn1 -- S1/RConn1

== system Isooffboard_SSC/DAB2/S3 ==
  g : Inport
  Diode : fl_lib/Electrical/Electrical Elements/Diode  Vf=1e-3 V  Ron=1e-2 Ohm  Goff=1e-5 1/Ohm  i_specify=off  i_priority=None  i=0 A  i_nominal_specify=off  i_nominal_value=1  i_nominal_unit=A  v_specify=off  v_priority=None  v=0 V  v_nominal_specify=off  v_nominal_value=1  v_nominal_unit=V
  S1 : fl_lib/Electrical/Electrical Elements/Switch  R_closed=0.1 Ohm  G_open=1e-5 1/Ohm  Threshold=0.5  i_specify=off  i_priority=None  i=0 A  i_nominal_specify=off  i_nominal_value=1  i_nominal_unit=A  v_specify=off  v_priority=None  v=0 V  v_nominal_specify=off  v_nominal_value=1  v_nominal_unit=V
  Simulink-PS Converter : nesl_utility/Simulink-PS Converter  PhysicalDomain=network_engine_domain  SubClassName=ps_input  LeftPortType=input  RightPortType=output  PseudoPeriodic=off  Frequencies=[]  NoiseDistribution=none  NoiseParameters=[]  Unit=1  AffineConversion=off  FilteringAndDerivatives=zero  SimscapeFilterOrder=1  InputFilterTimeConstant=0.001  UdotUserProvided=0
  + : PMIOPort  Side=Left
  - : PMIOPort  Port=2  Side=Right
  wires:
  g/1 -> Simulink-PS Converter/1
  connections:
  Simulink-PS Converter/RConn1 -- S1/RConn1
  S1/LConn1 -- +/RConn1 -- Diode/RConn1
  Diode/LConn1 -- -/RConn1 -- S1/RConn2

== system Isooffboard_SSC/DAB2/S4 ==
  g : Inport
  Diode : fl_lib/Electrical/Electrical Elements/Diode  Vf=1e-3 V  Ron=1e-2 Ohm  Goff=1e-5 1/Ohm  i_specify=off  i_priority=None  i=0 A  i_nominal_specify=off  i_nominal_value=1  i_nominal_unit=A  v_specify=off  v_priority=None  v=0 V  v_nominal_specify=off  v_nominal_value=1  v_nominal_unit=V
  S1 : fl_lib/Electrical/Electrical Elements/Switch  R_closed=0.1 Ohm  G_open=1e-5 1/Ohm  Threshold=0.5  i_specify=off  i_priority=None  i=0 A  i_nominal_specify=off  i_nominal_value=1  i_nominal_unit=A  v_specify=off  v_priority=None  v=0 V  v_nominal_specify=off  v_nominal_value=1  v_nominal_unit=V
  Simulink-PS Converter : nesl_utility/Simulink-PS Converter  PhysicalDomain=network_engine_domain  SubClassName=ps_input  LeftPortType=input  RightPortType=output  PseudoPeriodic=off  Frequencies=[]  NoiseDistribution=none  NoiseParameters=[]  Unit=1  AffineConversion=off  FilteringAndDerivatives=zero  SimscapeFilterOrder=1  InputFilterTimeConstant=0.001  UdotUserProvided=0
  + : PMIOPort  Side=Left
  - : PMIOPort  Port=2  Side=Right
  wires:
  g/1 -> Simulink-PS Converter/1
  connections:
  S1/RConn2 -- -/RConn1 -- Diode/LConn1
  Diode/RConn1 -- +/RConn1 -- S1/LConn1
  Simulink-PS Converter/RConn1 -- S1/RConn1

== system Isooffboard_SSC/DAB3/S1 ==
  g : Inport
  Diode : fl_lib/Electrical/Electrical Elements/Diode  Vf=1e-3 V  Ron=1e-2 Ohm  Goff=1e-5 1/Ohm  i_specify=off  i_priority=None  i=0 A  i_nominal_specify=off  i_nominal_value=1  i_nominal_unit=A  v_specify=off  v_priority=None  v=0 V  v_nominal_specify=off  v_nominal_value=1  v_nominal_unit=V
  S1 : fl_lib/Electrical/Electrical Elements/Switch  R_closed=0.1 Ohm  G_open=1e-5 1/Ohm  Threshold=0.5  i_specify=off  i_priority=None  i=0 A  i_nominal_specify=off  i_nominal_value=1  i_nominal_unit=A  v_specify=off  v_priority=None  v=0 V  v_nominal_specify=off  v_nominal_value=1  v_nominal_unit=V
  Simulink-PS Converter : nesl_utility/Simulink-PS Converter  PhysicalDomain=network_engine_domain  SubClassName=ps_input  LeftPortType=input  RightPortType=output  PseudoPeriodic=off  Frequencies=[]  NoiseDistribution=none  NoiseParameters=[]  Unit=1  AffineConversion=off  FilteringAndDerivatives=zero  SimscapeFilterOrder=1  InputFilterTimeConstant=0.001  UdotUserProvided=0
  + : PMIOPort  Side=Left
  - : PMIOPort  Port=2  Side=Right
  wires:
  g/1 -> Simulink-PS Converter/1
  connections:
  S1/RConn2 -- -/RConn1 -- Diode/LConn1
  Diode/RConn1 -- +/RConn1 -- S1/LConn1
  Simulink-PS Converter/RConn1 -- S1/RConn1

== system Isooffboard_SSC/DAB3/S2 ==
  g : Inport
  Diode : fl_lib/Electrical/Electrical Elements/Diode  Vf=1e-3 V  Ron=1e-2 Ohm  Goff=1e-5 1/Ohm  i_specify=off  i_priority=None  i=0 A  i_nominal_specify=off  i_nominal_value=1  i_nominal_unit=A  v_specify=off  v_priority=None  v=0 V  v_nominal_specify=off  v_nominal_value=1  v_nominal_unit=V
  S1 : fl_lib/Electrical/Electrical Elements/Switch  R_closed=0.1 Ohm  G_open=1e-5 1/Ohm  Threshold=0.5  i_specify=off  i_priority=None  i=0 A  i_nominal_specify=off  i_nominal_value=1  i_nominal_unit=A  v_specify=off  v_priority=None  v=0 V  v_nominal_specify=off  v_nominal_value=1  v_nominal_unit=V
  Simulink-PS Converter : nesl_utility/Simulink-PS Converter  PhysicalDomain=network_engine_domain  SubClassName=ps_input  LeftPortType=input  RightPortType=output  PseudoPeriodic=off  Frequencies=[]  NoiseDistribution=none  NoiseParameters=[]  Unit=1  AffineConversion=off  FilteringAndDerivatives=zero  SimscapeFilterOrder=1  InputFilterTimeConstant=0.001  UdotUserProvided=0
  + : PMIOPort  Side=Left
  - : PMIOPort  Port=2  Side=Right
  wires:
  g/1 -> Simulink-PS Converter/1
  connections:
  Simulink-PS Converter/RConn1 -- S1/RConn1
  S1/LConn1 -- +/RConn1 -- Diode/RConn1
  Diode/LConn1 -- -/RConn1 -- S1/RConn2

== system Isooffboard_SSC/DAB3/S3 ==
  g : Inport
  Diode : fl_lib/Electrical/Electrical Elements/Diode  Vf=1e-3 V  Ron=1e-2 Ohm  Goff=1e-5 1/Ohm  i_specify=off  i_priority=None  i=0 A  i_nominal_specify=off  i_nominal_value=1  i_nominal_unit=A  v_specify=off  v_priority=None  v=0 V  v_nominal_specify=off  v_nominal_value=1  v_nominal_unit=V
  S1 : fl_lib/Electrical/Electrical Elements/Switch  R_closed=0.1 Ohm  G_open=1e-5 1/Ohm  Threshold=0.5  i_specify=off  i_priority=None  i=0 A  i_nominal_specify=off  i_nominal_value=1  i_nominal_unit=A  v_specify=off  v_priority=None  v=0 V  v_nominal_specify=off  v_nominal_value=1  v_nominal_unit=V
  Simulink-PS Converter : nesl_utility/Simulink-PS Converter  PhysicalDomain=network_engine_domain  SubClassName=ps_input  LeftPortType=input  RightPortType=output  PseudoPeriodic=off  Frequencies=[]  NoiseDistribution=none  NoiseParameters=[]  Unit=1  AffineConversion=off  FilteringAndDerivatives=zero  SimscapeFilterOrder=1  InputFilterTimeConstant=0.001  UdotUserProvided=0
  + : PMIOPort  Side=Left
  - : PMIOPort  Port=2  Side=Right
  wires:
  g/1 -> Simulink-PS Converter/1
  connections:
  S1/RConn2 -- -/RConn1 -- Diode/LConn1
  Diode/RConn1 -- +/RConn1 -- S1/LConn1
  Simulink-PS Converter/RConn1 -- S1/RConn1

== system Isooffboard_SSC/DAB3/S4 ==
  g : Inport
  Diode : fl_lib/Electrical/Electrical Elements/Diode  Vf=1e-3 V  Ron=1e-2 Ohm  Goff=1e-5 1/Ohm  i_specify=off  i_priority=None  i=0 A  i_nominal_specify=off  i_nominal_value=1  i_nominal_unit=A  v_specify=off  v_priority=None  v=0 V  v_nominal_specify=off  v_nominal_value=1  v_nominal_unit=V
  S1 : fl_lib/Electrical/Electrical Elements/Switch  R_closed=0.1 Ohm  G_open=1e-5 1/Ohm  Threshold=0.5  i_specify=off  i_priority=None  i=0 A  i_nominal_specify=off  i_nominal_value=1  i_nominal_unit=A  v_specify=off  v_priority=None  v=0 V  v_nominal_specify=off  v_nominal_value=1  v_nominal_unit=V
  Simulink-PS Converter : nesl_utility/Simulink-PS Converter  PhysicalDomain=network_engine_domain  SubClassName=ps_input  LeftPortType=input  RightPortType=output  PseudoPeriodic=off  Frequencies=[]  NoiseDistribution=none  NoiseParameters=[]  Unit=1  AffineConversion=off  FilteringAndDerivatives=zero  SimscapeFilterOrder=1  InputFilterTimeConstant=0.001  UdotUserProvided=0
  + : PMIOPort  Side=Left
  - : PMIOPort  Port=2  Side=Right
  wires:
  g/1 -> Simulink-PS Converter/1
  connections:
  Simulink-PS Converter/RConn1 -- S1/RConn1
  S1/LConn1 -- +/RConn1 -- Diode/RConn1
  Diode/LConn1 -- -/RConn1 -- S1/RConn2

== system Isooffboard_SSC/Front End/S1 ==
  g : Inport
  Diode : fl_lib/Electrical/Electrical Elements/Diode  Vf=1e-3 V  Ron=1e-2 Ohm  Goff=1e-5 1/Ohm  i_specify=off  i_priority=None  i=0 A  i_nominal_specify=off  i_nominal_value=1  i_nominal_unit=A  v_specify=off  v_priority=None  v=0 V  v_nominal_specify=off  v_nominal_value=1  v_nominal_unit=V
  S1 : fl_lib/Electrical/Electrical Elements/Switch  R_closed=0.1 Ohm  G_open=1e-5 1/Ohm  Threshold=0.5  i_specify=off  i_priority=None  i=0 A  i_nominal_specify=off  i_nominal_value=1  i_nominal_unit=A  v_specify=off  v_priority=None  v=0 V  v_nominal_specify=off  v_nominal_value=1  v_nominal_unit=V
  Simulink-PS Converter : nesl_utility/Simulink-PS Converter  PhysicalDomain=network_engine_domain  SubClassName=ps_input  LeftPortType=input  RightPortType=output  PseudoPeriodic=off  Frequencies=[]  NoiseDistribution=none  NoiseParameters=[]  Unit=1  AffineConversion=off  FilteringAndDerivatives=zero  SimscapeFilterOrder=1  InputFilterTimeConstant=0.001  UdotUserProvided=0
  + : PMIOPort  Side=Left
  - : PMIOPort  Port=2  Side=Right
  wires:
  g/1 -> Simulink-PS Converter/1
  connections:
  S1/RConn2 -- -/RConn1 -- Diode/LConn1
  Diode/RConn1 -- +/RConn1 -- S1/LConn1
  Simulink-PS Converter/RConn1 -- S1/RConn1

== system Isooffboard_SSC/Front End/S2 ==
  g : Inport
  Diode : fl_lib/Electrical/Electrical Elements/Diode  Vf=1e-3 V  Ron=1e-2 Ohm  Goff=1e-5 1/Ohm  i_specify=off  i_priority=None  i=0 A  i_nominal_specify=off  i_nominal_value=1  i_nominal_unit=A  v_specify=off  v_priority=None  v=0 V  v_nominal_specify=off  v_nominal_value=1  v_nominal_unit=V
  S1 : fl_lib/Electrical/Electrical Elements/Switch  R_closed=0.1 Ohm  G_open=1e-5 1/Ohm  Threshold=0.5  i_specify=off  i_priority=None  i=0 A  i_nominal_specify=off  i_nominal_value=1  i_nominal_unit=A  v_specify=off  v_priority=None  v=0 V  v_nominal_specify=off  v_nominal_value=1  v_nominal_unit=V
  Simulink-PS Converter : nesl_utility/Simulink-PS Converter  PhysicalDomain=network_engine_domain  SubClassName=ps_input  LeftPortType=input  RightPortType=output  PseudoPeriodic=off  Frequencies=[]  NoiseDistribution=none  NoiseParameters=[]  Unit=1  AffineConversion=off  FilteringAndDerivatives=zero  SimscapeFilterOrder=1  InputFilterTimeConstant=0.001  UdotUserProvided=0
  + : PMIOPort  Side=Left
  - : PMIOPort  Port=2  Side=Right
  wires:
  g/1 -> Simulink-PS Converter/1
  connections:
  Simulink-PS Converter/RConn1 -- S1/RConn1
  S1/LConn1 -- +/RConn1 -- Diode/RConn1
  Diode/LConn1 -- -/RConn1 -- S1/RConn2

== system Isooffboard_SSC/Front End/S3 ==
  g : Inport
  Diode : fl_lib/Electrical/Electrical Elements/Diode  Vf=1e-3 V  Ron=1e-2 Ohm  Goff=1e-5 1/Ohm  i_specify=off  i_priority=None  i=0 A  i_nominal_specify=off  i_nominal_value=1  i_nominal_unit=A  v_specify=off  v_priority=None  v=0 V  v_nominal_specify=off  v_nominal_value=1  v_nominal_unit=V
  S1 : fl_lib/Electrical/Electrical Elements/Switch  R_closed=0.1 Ohm  G_open=1e-5 1/Ohm  Threshold=0.5  i_specify=off  i_priority=None  i=0 A  i_nominal_specify=off  i_nominal_value=1  i_nominal_unit=A  v_specify=off  v_priority=None  v=0 V  v_nominal_specify=off  v_nominal_value=1  v_nominal_unit=V
  Simulink-PS Converter : nesl_utility/Simulink-PS Converter  PhysicalDomain=network_engine_domain  SubClassName=ps_input  LeftPortType=input  RightPortType=output  PseudoPeriodic=off  Frequencies=[]  NoiseDistribution=none  NoiseParameters=[]  Unit=1  AffineConversion=off  FilteringAndDerivatives=zero  SimscapeFilterOrder=1  InputFilterTimeConstant=0.001  UdotUserProvided=0
  + : PMIOPort  Side=Left
  - : PMIOPort  Port=2  Side=Right
  wires:
  g/1 -> Simulink-PS Converter/1
  connections:
  S1/RConn2 -- -/RConn1 -- Diode/LConn1
  Diode/RConn1 -- +/RConn1 -- S1/LConn1
  Simulink-PS Converter/RConn1 -- S1/RConn1

== system Isooffboard_SSC/Front End/S4 ==
  g : Inport
  Diode : fl_lib/Electrical/Electrical Elements/Diode  Vf=1e-3 V  Ron=1e-2 Ohm  Goff=1e-5 1/Ohm  i_specify=off  i_priority=None  i=0 A  i_nominal_specify=off  i_nominal_value=1  i_nominal_unit=A  v_specify=off  v_priority=None  v=0 V  v_nominal_specify=off  v_nominal_value=1  v_nominal_unit=V
  S1 : fl_lib/Electrical/Electrical Elements/Switch  R_closed=0.1 Ohm  G_open=1e-5 1/Ohm  Threshold=0.5  i_specify=off  i_priority=None  i=0 A  i_nominal_specify=off  i_nominal_value=1  i_nominal_unit=A  v_specify=off  v_priority=None  v=0 V  v_nominal_specify=off  v_nominal_value=1  v_nominal_unit=V
  Simulink-PS Converter : nesl_utility/Simulink-PS Converter  PhysicalDomain=network_engine_domain  SubClassName=ps_input  LeftPortType=input  RightPortType=output  PseudoPeriodic=off  Frequencies=[]  NoiseDistribution=none  NoiseParameters=[]  Unit=1  AffineConversion=off  FilteringAndDerivatives=zero  SimscapeFilterOrder=1  InputFilterTimeConstant=0.001  UdotUserProvided=0
  + : PMIOPort  Side=Left
  - : PMIOPort  Port=2  Side=Right
  wires:
  g/1 -> Simulink-PS Converter/1
  connections:
  Simulink-PS Converter/RConn1 -- S1/RConn1
  S1/LConn1 -- +/RConn1 -- Diode/RConn1
  Diode/LConn1 -- -/RConn1 -- S1/RConn2

== system Isooffboard_SSC/Front End/S5 ==
  g : Inport
  Diode : fl_lib/Electrical/Electrical Elements/Diode  Vf=1e-3 V  Ron=1e-2 Ohm  Goff=1e-5 1/Ohm  i_specify=off  i_priority=None  i=0 A  i_nominal_specify=off  i_nominal_value=1  i_nominal_unit=A  v_specify=off  v_priority=None  v=0 V  v_nominal_specify=off  v_nominal_value=1  v_nominal_unit=V
  S1 : fl_lib/Electrical/Electrical Elements/Switch  R_closed=0.1 Ohm  G_open=1e-5 1/Ohm  Threshold=0.5  i_specify=off  i_priority=None  i=0 A  i_nominal_specify=off  i_nominal_value=1  i_nominal_unit=A  v_specify=off  v_priority=None  v=0 V  v_nominal_specify=off  v_nominal_value=1  v_nominal_unit=V
  Simulink-PS Converter : nesl_utility/Simulink-PS Converter  PhysicalDomain=network_engine_domain  SubClassName=ps_input  LeftPortType=input  RightPortType=output  PseudoPeriodic=off  Frequencies=[]  NoiseDistribution=none  NoiseParameters=[]  Unit=1  AffineConversion=off  FilteringAndDerivatives=zero  SimscapeFilterOrder=1  InputFilterTimeConstant=0.001  UdotUserProvided=0
  + : PMIOPort  Side=Left
  - : PMIOPort  Port=2  Side=Right
  wires:
  g/1 -> Simulink-PS Converter/1
  connections:
  S1/RConn2 -- -/RConn1 -- Diode/LConn1
  Diode/RConn1 -- +/RConn1 -- S1/LConn1
  Simulink-PS Converter/RConn1 -- S1/RConn1

== system Isooffboard_SSC/Front End/S6 ==
  g : Inport
  Diode : fl_lib/Electrical/Electrical Elements/Diode  Vf=1e-3 V  Ron=1e-2 Ohm  Goff=1e-5 1/Ohm  i_specify=off  i_priority=None  i=0 A  i_nominal_specify=off  i_nominal_value=1  i_nominal_unit=A  v_specify=off  v_priority=None  v=0 V  v_nominal_specify=off  v_nominal_value=1  v_nominal_unit=V
  S1 : fl_lib/Electrical/Electrical Elements/Switch  R_closed=0.1 Ohm  G_open=1e-5 1/Ohm  Threshold=0.5  i_specify=off  i_priority=None  i=0 A  i_nominal_specify=off  i_nominal_value=1  i_nominal_unit=A  v_specify=off  v_priority=None  v=0 V  v_nominal_specify=off  v_nominal_value=1  v_nominal_unit=V
  Simulink-PS Converter : nesl_utility/Simulink-PS Converter  PhysicalDomain=network_engine_domain  SubClassName=ps_input  LeftPortType=input  RightPortType=output  PseudoPeriodic=off  Frequencies=[]  NoiseDistribution=none  NoiseParameters=[]  Unit=1  AffineConversion=off  FilteringAndDerivatives=zero  SimscapeFilterOrder=1  InputFilterTimeConstant=0.001  UdotUserProvided=0
  + : PMIOPort  Side=Left
  - : PMIOPort  Port=2  Side=Right
  wires:
  g/1 -> Simulink-PS Converter/1
  connections:
  Simulink-PS Converter/RConn1 -- S1/RConn1
  S1/LConn1 -- +/RConn1 -- Diode/RConn1
  Diode/LConn1 -- -/RConn1 -- S1/RConn2

== matlab function Isooffboard_SSC/Subsystem3/MATLAB Function ==
  data: u input; y output
function y = fcn(u)
persistent t;
if isempty (t)
t=0;
end
frequency = u*105310; %105310 
t=t+0.0000001;

y = (sawtooth(2 * pi * frequency * t, 0.5)+1)/2;

== matlab function Isooffboard_SSC/Subsystem5/MATLAB Function ==
  data: u input; y output
function y = fcn(u)
persistent t;
if isempty (t)
t=0;
end
frequency = u*105310; %105310 
t=t+0.0000001;

y = (sawtooth(2 * pi * frequency * t, 0.5)+1)/2;
